simulink model "ForEach3"  (R2017b)
settings: Solver=ode3  StartTime=0.0  StopTime=10.0  FixedStep=0.200000  RelTol=1e-3  EnableMultiTasking=on
settings Model: Creator=hbourbou  LastModifiedBy=hbourbou
settings DataIOCC: LimitDataPoints=on  SaveFormat=Structure
settings OptimizationCC: LifeSpan=inf
settings DebuggingCC: SFUnexpectedBacktrackingDiag=warning  SFNoUnconditionalDefaultTransitionDiag=warning  SFExecutionAtInitializationDiag=none
settings HardwareCC: ProdBitPerPointer=32  ProdBitPerSizeT=32  ProdBitPerPtrDiffT=32  ProdLargestAtomicFloat=None  ProdIntDivRoundTo=Undefined  ProdEndianess=Unspecified  ProdWordSize=32  ProdHWDeviceType=32-bit Generic
settings ModelReferenceCC: PropagateSignalLabelsOutOfModel=off
settings CodeAppCC: StateflowObjectComments=on
settings GRTTargetCC: TargetLangStandard=C89/C90 (ANSI)  GeneratePreprocessorConditionals=Disable all
settings ConfigComp: CovMetricSettings=dw  CovHtmlReporting=on  CovSaveCumulativeToWorkspaceVar=on  CovSaveSingleToWorkspaceVar=on  CovExternalEMLEnable=off

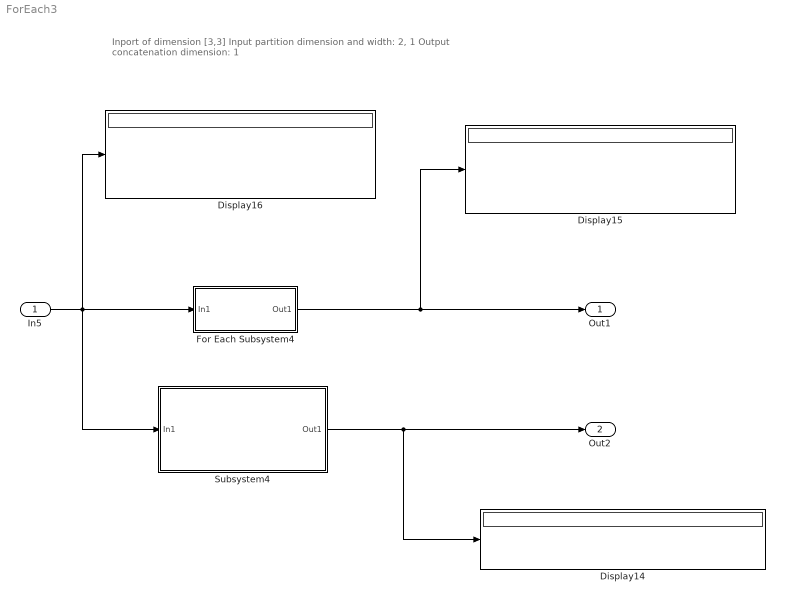
== system ForEach3 ==
  note: Inport of dimension [3,3]
      | Input partition dimension and width: 2, 1
      | Output concatenation dimension: 1
  In5 : Inport  PortDimensions=[3 3]
  Display14 : Display
  Display15 : Display
  Display16 : Display
  For Each Subsystem4 : Subsystem
  Subsystem4 : Subsystem
  Out1 : Outport
  Out2 : Outport  Port=2
  wires:
  In5/1 -> Display16/1, For Each Subsystem4/1(In1), Subsystem4/1(In1)
  For Each Subsystem4/1(Out1) -> Out1/1, Display15/1
  Subsystem4/1(Out1) -> Out2/1, Display14/1

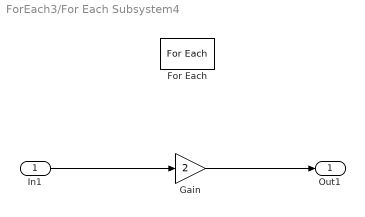
== system ForEach3/For Each Subsystem4 ==
  In1 : Inport  Partition=on  PartitionDimension=2  PartitionWidth=1  PartitionOffset=0
  For Each : ForEach  DisableCoverage=on  IndexMode=One-based
  Gain : Gain  Gain=2
  Out1 : Outport  ConcatenationDimension=1
  wires:
  Gain/1 -> Out1/1
  In1/1 -> Gain/1

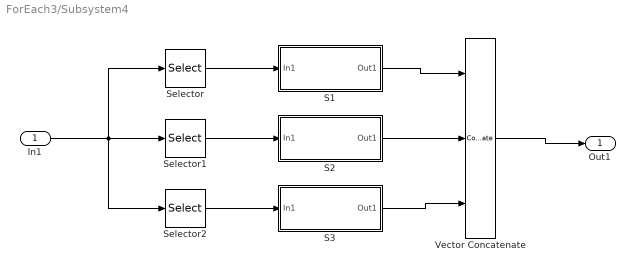
== system ForEach3/Subsystem4 ==
  In1 : Inport
  S1 : Subsystem
  S2 : Subsystem
  S3 : Subsystem
  Selector : Selector  NumberOfDimensions=2  InputPortWidth=3  IndexOptions=Select all,Index vector (dialog)  Indices=1,1  OutputSizes=1,1
  Selector1 : Selector  NumberOfDimensions=2  InputPortWidth=3  IndexOptions=Select all,Index vector (dialog)  Indices=2,2  OutputSizes=1,1
  Selector2 : Selector  NumberOfDimensions=2  InputPortWidth=3  IndexOptions=Select all,Index vector (dialog)  Indices=3,3  OutputSizes=1,1
  Vector Concatenate : Concatenate  NumInputs=3  Mode=Multidimensional array
  Out1 : Outport
  wires:
  S1/1(Out1) -> Vector Concatenate/1
  S3/1(Out1) -> Vector Concatenate/3
  S2/1(Out1) -> Vector Concatenate/2
  Selector/1 -> S1/1(In1)
  Vector Concatenate/1 -> Out1/1
  Selector2/1 -> S3/1(In1)
  Selector1/1 -> S2/1(In1)
  In1/1 -> Selector2/1, Selector1/1, Selector/1

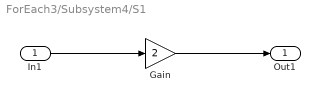
== system ForEach3/Subsystem4/S1 ==
  In1 : Inport
  Gain : Gain  Gain=2
  Out1 : Outport
  wires:
  In1/1 -> Gain/1
  Gain/1 -> Out1/1

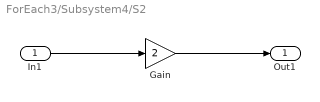
== system ForEach3/Subsystem4/S2 ==
  In1 : Inport
  Gain : Gain  Gain=2
  Out1 : Outport
  wires:
  In1/1 -> Gain/1
  Gain/1 -> Out1/1

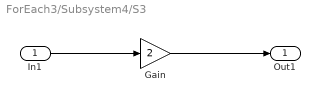
== system ForEach3/Subsystem4/S3 ==
  In1 : Inport
  Gain : Gain  Gain=2
  Out1 : Outport
  wires:
  In1/1 -> Gain/1
  Gain/1 -> Out1/1
